simulink model "york199"  (Simulink 7.2)
settings: Solver=ode45  StartTime=0.0  StopTime=10.0  RelTol=1e-3
settings Model: Creator=alesch  LastModifiedBy=alesch

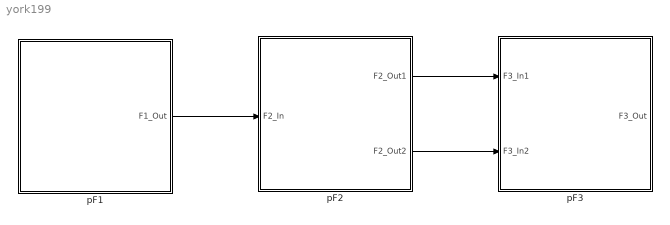
== system york199 ==
  pF1 : Subsystem
  pF2 : Subsystem
  pF3 : Subsystem
  wires:
  pF1/1(F1_Out) -> pF2/1(F2_In)
  pF2/1(F2_Out1) -> pF3/1(F3_In1)
  pF2/2(F2_Out2) -> pF3/2(F3_In2)

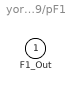
== system york199/pF1 ==
  F1_Out : Outport

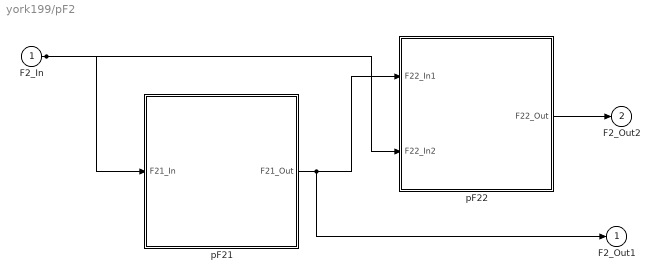
== system york199/pF2 ==
  F2_In : Inport
  pF21 : Subsystem
  pF22 : Subsystem
  F2_Out1 : Outport
  F2_Out2 : Outport  Port=2
  wires:
  F2_In/1 -> pF21/1(F21_In), pF22/2(F22_In2)
  pF21/1(F21_Out) -> F2_Out1/1, pF22/1(F22_In1)
  pF22/1(F22_Out) -> F2_Out2/1

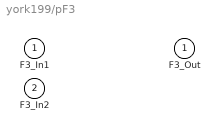
== system york199/pF3 ==
  F3_In1 : Inport
  F3_In2 : Inport  Port=2
  F3_Out : Outport

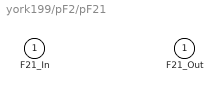
== system york199/pF2/pF21 ==
  F21_In : Inport
  F21_Out : Outport

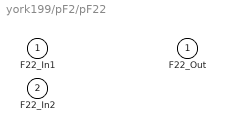
== system york199/pF2/pF22 ==
  F22_In1 : Inport
  F22_In2 : Inport  Port=2
  F22_Out : Outport
